simulink model "bldc_cc_2020a"  (R2020a)
settings: Solver=VariableStepAuto  StartTime=0.0  StopTime=10  RelTol=1e-3
undefined symbols (not defined in the file or in its folder): Ion, Lithium
libraries: spsMosfetLib x6, spsSeriesRLCBranchLib x3, simulink x3, spsBatteryLib x1, spsPermanentMagnetSynchronousMachineLib x1, spspowerguiLib x1
settings Model: Creator=Deepak  LastModifiedBy=giulio
settings SFSimCC: CustomCodeUndefinedFunction=UseInterfaceOnly

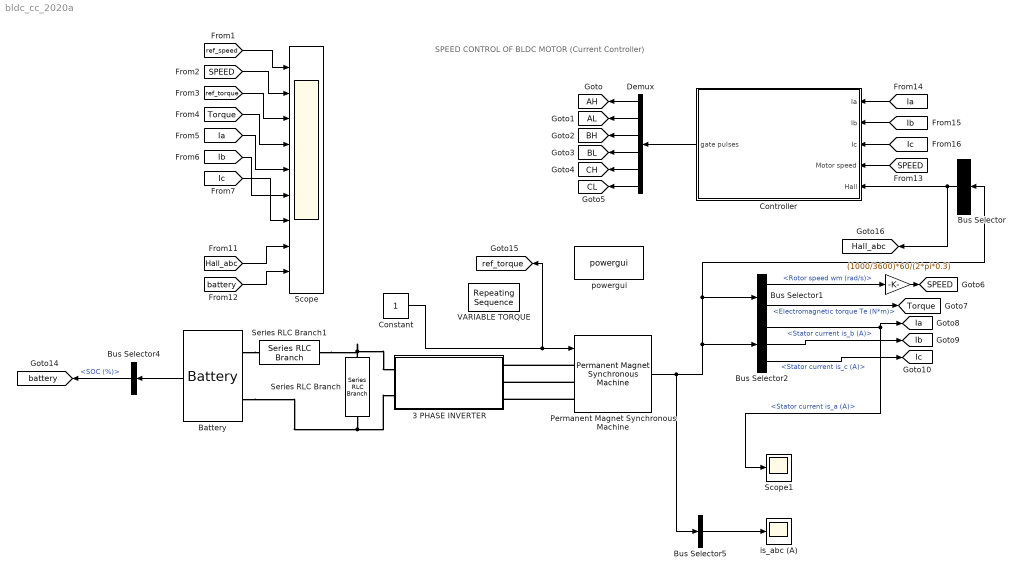
== system bldc_cc_2020a ==
  note: SPEED CONTROL OF BLDC MOTOR (Current Controller)
  " " : Gain  Gain=(1000/3600)*60/(2*pi*0.3)
  3 PHASE INVERTER : Subsystem
  Battery : spsBatteryLib/Battery  BatType=Lithium-Ion  ShowTempParam=off  ThermalPreset=no  ShowAgeParam=off  NomV=12  NomQ=80  SOC=60  Batt_Tr=30  PresetModel=off  MaxQ=84  MinV=36  FullV=56.818272  Dis_rate=27.82608  R=0.006  Normal_OP=57.87524  expZone=[54.89208 3.144344]  current=[1.5 3]  Units=Ampere-hour  Tci=20  NomT=20  T2=-30  MaxQ2=4.8  FullV2=7.1  Normal_OP2=5.655  expZone2="[6.58           1]"  Rca=0.6  ti=2000  Dp=0  Neq0=0  Tsim=1e6  Ta1=25  Qeol=5.4*0.9  Reol=0.013333*1.2  Char_age=[2.3478, 3]  Dis_age=[2.3478, 10]  N1=1500  N2=10500  N3=1000  N4=1400  Ta2=45  N5=950
  Bus Selector : BusSelector  OutputSignals=Hall effect signal h_a,Hall effect signal h_b,Hall effect signal h_c  OutputAsBus=on
  Bus Selector1 : BusSelector  OutputSignals=Rotor speed wm (rad/s),Electromagnetic torque Te (N*m)
  Bus Selector2 : BusSelector  OutputSignals=Stator current is_a (A),Stator current is_b (A),Stator current is_c (A)
  Bus Selector4 : BusSelector  OutputSignals=SOC (%)
  Bus Selector5 : BusSelector  OutputSignals=Stator current is_a (A),Stator current is_b (A),Stator current is_c (A)  OutputAsBus=on
  Constant : Constant
  Controller : Subsystem
  Demux : Demux  Outputs=6
  Permanent Magnet Synchronous Machine : spsPermanentMagnetSynchronousMachineLib/Permanent Magnet Synchronous Machine  NbPhases=3  FluxDistribution=Sinusoidal  RotorType=Round  MechanicalLoad=Torque Tm  PresetModel=No  ShowDetailedParameters=on  MeasurementBus=off  Resistance=2.875  Inductance=8.5e-3  dqInductances=[8.5e-3,8.5e-3]  La=0.00153  MachineConstant=Flux linkage established by magnets (V.s)  Flux=0.175  VoltageCst=126.966  TorqueCst=1.05  Flat=120  Mechanical=[ 0.8e-3, 0 4]  PolePairs=4  InitialConditions=[0,0, 0,0]  InitialConditions5ph=[0 0 0 0 0 0]  RefAngle=90 degrees behind phase A axis (modified Park)  IterativeDiscreteModel=Trapezoidal non iterative  TsBlock=-1  TsPowergui=0
  Scope : Scope  NumInputPorts=9
  Scope1 : Scope
  Series RLC Branch : spsSeriesRLCBranchLib/Series RLC Branch  LConnTagsString=__new0  RConnTagsString=__new0  BranchType=C  Resistance=1  Inductance=1e-3  SetiL0=off  InitialCurrent=0  Capacitance=75e-3  Setx0=off  InitialVoltage=0  Measurements=None
  Series RLC Branch1 : spsSeriesRLCBranchLib/Series RLC Branch  LConnTagsString=__new0  RConnTagsString=__new0  BranchType=RL  Resistance=1  Inductance=1e-3  SetiL0=off  InitialCurrent=0  Capacitance=75e-3  Setx0=off  InitialVoltage=0  Measurements=None
  VARIABLE TORQUE : simulink/Sources/Repeating Sequence  rep_seq_t=[0 1 2 3 4 5 6 7 8 9 10 11 12 13]  rep_seq_y=[3 3 3 3 5 5 5 -2 -2 -2 1 1 1 1 ]
  is_abc (A) : Scope
  powergui : spspowerguiLib/powergui  Priority=1  SimulationMode=Discrete  SampleTime=10e-6  frequency=60  Iterations=50  frequencyindice=0  Pbase=100e6  ErrMax=1e-4  UnitsV=kV  UnitsW=MW  buscounter=0  FunctionMessages=off  echomessages=off  EnableUseOfTLC=off  CurrentSourceSwitches=off  DisableSnubberDevices=off  DisableRonSwitches=off  DisableVfSwitches=off  DisplayEquations=off  AutomaticDiscreteSolvers=off  SolverType=Tustin/Backward Euler (TBE)  Interpol=off  ExternalGateDelay=off  methode=off  Ts=100  x0status=blocks  SPID=on  SwTol=0  HookPort=off  NonlinearTolerance=0  nMaxIteration=15  ContinueOnMaxIteration=off  RestoreLinks=warning  ResistiveCurrentMeasurement=off  Frange=[0:2:500]  Ylog=off  Xlog=on  ShowGrid=off  save=off  variable=ZData  structure=0  ZoomFFT=off  StartTime=0.0  cycles=1  DisplayStyle=1  fundamental=60  FreqAxis=off  MaxFrequency=1000  frequencyindicesteady=1  RmsSteady=1  display=off
  tag scope: AH=global, AL=global, BH=global, BL=global, CH=global, CL=global, Hall_abc=global, Ia=global, Ib=global, Ic=global, SPEED=global, Torque=global, battery=global, ref_torque=global
  wires:
  [SPEED] -> Scope/2
  [ref_torque] -> Scope/3
  [Ic] -> Scope/7
  Bus Selector2/2 -> [Ib]  "<Stator current is_b (A)>"
  [Hall_abc] -> Scope/8
  Demux/4 -> [BL]
  Demux/3 -> [BH]
  " "/1 -> [SPEED]
  [Ib] -> Scope/6
  [Ia] -> Scope/5
  Bus Selector2/3 -> [Ic]  "<Stator current is_c (A)>"
  [Torque] -> Scope/4
  Bus Selector1/1 -> " "/1  "<Rotor speed wm (rad/s)>"
  [battery] -> Scope/9
  Bus Selector1/2 -> [Torque]  "<Electromagnetic torque Te (N*m)>"
  [ref_speed] -> Scope/1
  Demux/5 -> [CH]
  Demux/1 -> [AH]
  Demux/6 -> [CL]
  Demux/2 -> [AL]
  Bus Selector2/1 -> Scope1/1, [Ia]  "<Stator current is_a (A)>"
  Bus Selector/1 -> Controller/5("Hall "), [Hall_abc]
  [SPEED] -> Controller/4(Motor speed)
  [Ia] -> Controller/1(Ia)
  [Ib] -> Controller/2(Ib)
  [Ic] -> Controller/3(Ic)
  Controller/1(gate pulses) -> Demux/1
  Battery/1 -> Bus Selector4/1
  Bus Selector4/1 -> [battery]  "<SOC (%)>"
  Constant/1 -> Permanent Magnet Synchronous Machine/1, [ref_torque]
  Bus Selector5/1 -> is_abc (A)/1
  Permanent Magnet Synchronous Machine/1 -> Bus Selector5/1, Bus Selector/1, Bus Selector1/1, Bus Selector2/1
  connections:
  Permanent Magnet Synchronous Machine/LConn2 -- 3 PHASE INVERTER/RConn2
  Permanent Magnet Synchronous Machine/LConn3 -- 3 PHASE INVERTER/RConn3
  Permanent Magnet Synchronous Machine/LConn1 -- 3 PHASE INVERTER/RConn1
  Battery/LConn2 -- Series RLC Branch/RConn1 -- 3 PHASE INVERTER/LConn2
  Series RLC Branch/LConn1 -- Series RLC Branch1/LConn1 -- 3 PHASE INVERTER/LConn1
  Battery/LConn1 -- Series RLC Branch1/RConn1

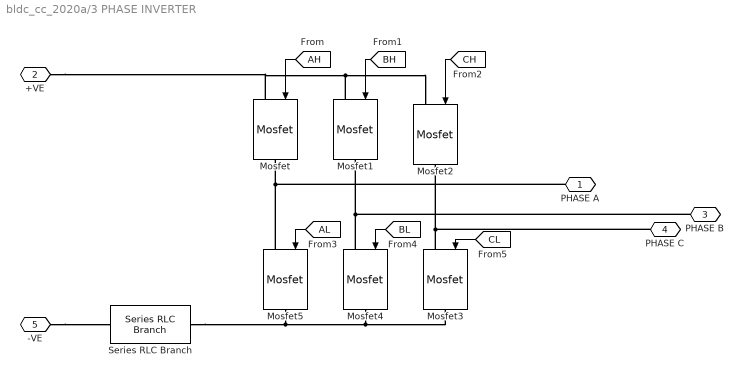
== system bldc_cc_2020a/3 PHASE INVERTER ==
  Mosfet{,1..5} (6 alike) : spsMosfetLib/Mosfet  Ron=0.1  Lon=0  Rd=0.01  Vfd=0  IC=0  Rs=1e5  Cs=inf  Measurements=off
  Series RLC Branch : spsSeriesRLCBranchLib/Series RLC Branch  LConnTagsString=__new0  RConnTagsString=__new0  BranchType=R  Resistance=1  Inductance=1e-3  SetiL0=off  InitialCurrent=0  Capacitance=1e-6  Setx0=off  InitialVoltage=0  Measurements=None
  PHASE A : PMIOPort  Side=Right
  +VE : PMIOPort  Port=2  Side=Left
  PHASE B : PMIOPort  Port=3  Side=Right
  PHASE C : PMIOPort  Port=4  Side=Right
  -VE : PMIOPort  Port=5  Side=Left
  wires:
  [AH] -> Mosfet/1
  [BH] -> Mosfet1/1
  [CH] -> Mosfet2/1
  [AL] -> Mosfet5/1
  [BL] -> Mosfet4/1
  [CL] -> Mosfet3/1
  connections:
  Mosfet5/LConn1 -- PHASE A/RConn1 -- Mosfet/RConn1
  PHASE B/RConn1 -- Mosfet4/LConn1 -- Mosfet1/RConn1
  Mosfet3/LConn1 -- Mosfet2/RConn1 -- PHASE C/RConn1
  Mosfet1/LConn1 -- Mosfet2/LConn1 -- Mosfet/LConn1 -- +VE/RConn1
  Mosfet5/RConn1 -- Series RLC Branch/RConn1 -- Mosfet4/RConn1 -- Mosfet3/RConn1
  -VE/RConn1 -- Series RLC Branch/LConn1

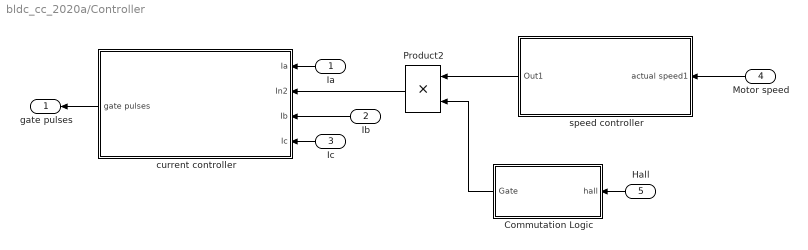
== system bldc_cc_2020a/Controller ==
  Ia : Inport
  Ib : Inport  Port=2
  Ic : Inport  Port=3
  Motor speed : Inport  Port=4
  "Hall " : Inport  Port=5
  Commutation Logic : Subsystem
  Product2 : Product  SaturateOnIntegerOverflow=on  OutDataTypeStr=Inherit: Same as first input
  current controller : Subsystem
  speed controller : Subsystem
  gate pulses : Outport  VectorParamsAs1DForOutWhenUnconnected=off
  wires:
  "Hall "/1 -> Commutation Logic/1("hall ")
  Commutation Logic/1(Gate) -> Product2/2
  current controller/1(gate pulses) -> gate pulses/1
  Ic/1 -> current controller/4(Ic)
  Ib/1 -> current controller/3(Ib)
  Ia/1 -> current controller/1(Ia)
  Product2/1 -> current controller/2(In2)
  Motor speed/1 -> speed controller/1(actual speed1)
  speed controller/1(Out1) -> Product2/1

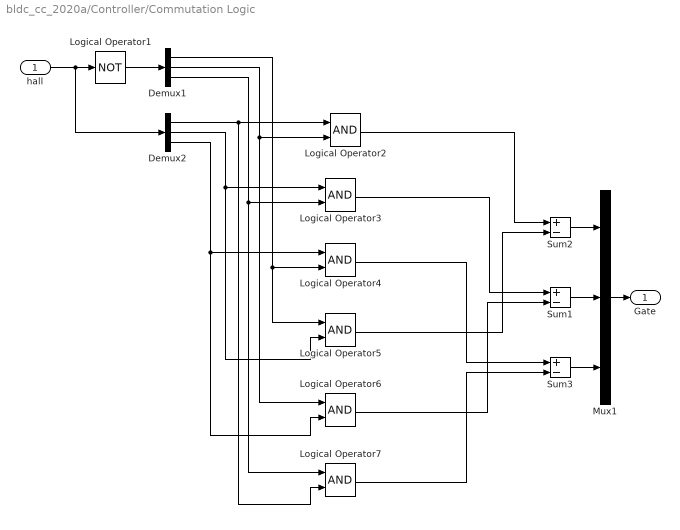
== system bldc_cc_2020a/Controller/Commutation Logic ==
  "hall " : Inport
  Demux1 : Demux  Outputs=3
  Demux2 : Demux  Outputs=3
  Logical Operator1 : Logic  Operator=NOT  AllPortsSameDT=off  OutDataTypeStr=boolean
  Logical Operator{2..7} (6 alike) : Logic  AllPortsSameDT=off  OutDataTypeStr=boolean
  Mux1 : Mux  Inputs=3
  Sum1 : Sum  Inputs=+-  OutDataTypeStr=double
  Sum2 : Sum  Inputs=+-  OutDataTypeStr=double
  Sum3 : Sum  Inputs=+-  OutDataTypeStr=double
  Gate : Outport  VectorParamsAs1DForOutWhenUnconnected=off
  wires:
  Demux2/1 -> Logical Operator7/2, Logical Operator2/1
  Demux1/3 -> Logical Operator7/1, Logical Operator3/2
  Demux2/2 -> Logical Operator3/1, Logical Operator5/2
  Sum1/1 -> Mux1/2
  Logical Operator3/1 -> Sum1/1
  "hall "/1 -> Logical Operator1/1, Demux2/1
  Demux1/2 -> Logical Operator6/1, Logical Operator2/2
  Logical Operator2/1 -> Sum2/1
  Logical Operator7/1 -> Sum3/2
  Logical Operator4/1 -> Sum3/1
  Demux1/1 -> Logical Operator4/2, Logical Operator5/1
  Logical Operator6/1 -> Sum1/2
  Logical Operator5/1 -> Sum2/2
  Sum3/1 -> Mux1/3
  Logical Operator1/1 -> Demux1/1
  Mux1/1 -> Gate/1
  Sum2/1 -> Mux1/1
  Demux2/3 -> Logical Operator4/1, Logical Operator6/2

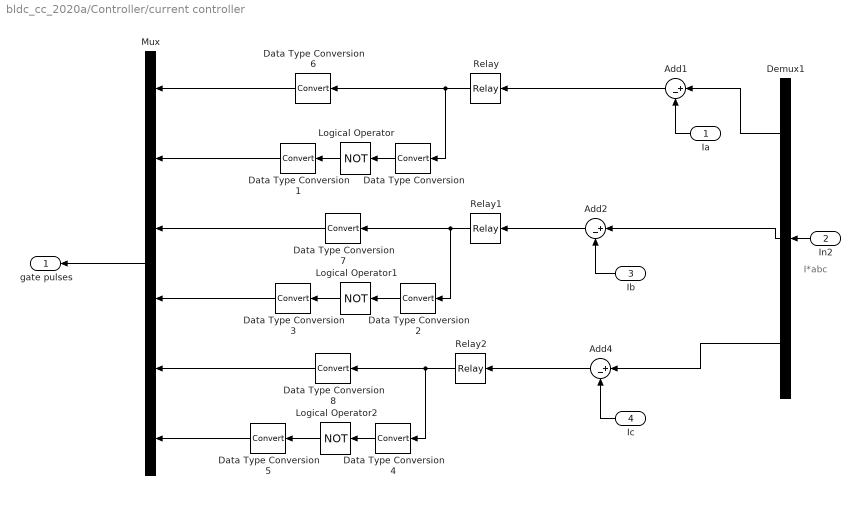
== system bldc_cc_2020a/Controller/current controller ==
  note: I*abc
  Ia : Inport
  In2 : Inport  Port=2
  Ib : Inport  Port=3
  Ic : Inport  Port=4
  Add1 : Sum  Inputs=|+-
  Add2 : Sum  Inputs=|+-
  Add4 : Sum  Inputs=|+-
  Data Type Conversion{,1..8} (9 alike) : DataTypeConversion  SaturateOnIntegerOverflow=on  RndMeth=Zero
  Demux1 : Demux  Outputs=3
      settings: DisplayOption=none
  Logical Operator : Logic  Operator=NOT  AllPortsSameDT=off  OutDataTypeStr=boolean
  Logical Operator1 : Logic  Operator=NOT  AllPortsSameDT=off  OutDataTypeStr=boolean
  Logical Operator2 : Logic  Operator=NOT  AllPortsSameDT=off  OutDataTypeStr=boolean
  Mux : Mux  Inputs=6
  Relay : Relay  OnSwitchValue=0.1  OffSwitchValue=-0.1
  Relay1 : Relay  OnSwitchValue=0.1  OffSwitchValue=-0.1
  Relay2 : Relay  OnSwitchValue=0.1  OffSwitchValue=-0.1
  gate pulses : Outport  VectorParamsAs1DForOutWhenUnconnected=off
  wires:
  Relay/1 -> Data Type Conversion6/1, Data Type Conversion/1
  Relay1/1 -> Data Type Conversion7/1, Data Type Conversion2/1
  Relay2/1 -> Data Type Conversion8/1, Data Type Conversion4/1
  Ib/1 -> Add2/2
  Mux/1 -> gate pulses/1
  Ic/1 -> Add4/2
  Data Type Conversion/1 -> Logical Operator/1
  Logical Operator/1 -> Data Type Conversion1/1
  Data Type Conversion1/1 -> Mux/2
  Logical Operator1/1 -> Data Type Conversion3/1
  Data Type Conversion3/1 -> Mux/4
  Data Type Conversion2/1 -> Logical Operator1/1
  Data Type Conversion5/1 -> Mux/6
  Logical Operator2/1 -> Data Type Conversion5/1
  Data Type Conversion4/1 -> Logical Operator2/1
  Demux1/2 -> Add2/1
  Demux1/3 -> Add4/1
  In2/1 -> Demux1/1
  Ia/1 -> Add1/2
  Demux1/1 -> Add1/1
  Add1/1 -> Relay/1
  Add2/1 -> Relay1/1
  Data Type Conversion6/1 -> Mux/1
  Data Type Conversion7/1 -> Mux/3
  Data Type Conversion8/1 -> Mux/5
  Add4/1 -> Relay2/1

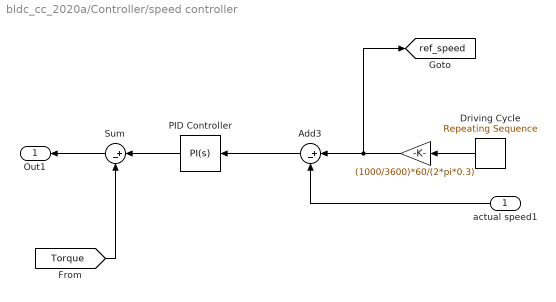
== system bldc_cc_2020a/Controller/speed controller ==
  actual speed1 : Inport
  " " : Gain  Gain=(1000/3600)*60/(2*pi*0.3)
  Add3 : Sum  Inputs=|+-
  Driving Cycle : simulink/Sources/Repeating Sequence  rep_seq_t=[0 1 2 3 4 5 6 7 8 9 10 11 11.0001 12 13]  rep_seq_y=[0 0 20 20 20 20 20 20 20 20 20 20 20 20 20]
  PID Controller : simulink/Continuous/PID Controller  Controller=PI  Form=Parallel  TimeDomain=Continuous-time  UseExternalTs=off  SampleTime=-1  IntegratorMethod=Forward Euler  FilterMethod=Forward Euler  ControllerParametersSource=internal  P=5  I=4.9  D=0  UseFilter=on  N=100  TunerSelectOption=Transfer Function Based (PID Tuner App)  InitialConditionSource=internal  InitialConditionForIntegrator=0  InitialConditionForFilter=0  DifferentiatorICPrevScaledInput=0  ExternalReset=none  TrackingMode=off  Kt=1  LimitOutput=off  UpperSaturationLimit=10  LowerSaturationLimit=0  LinearizeAsGain=on  AntiWindupMode=none  Kb=1  POutMin=[]  POutMax=[]  IOutMin=[]  IOutMax=[]  DOutMin=[]  DOutMax=[]  NOutMin=[]  NOutMax=[]  SumOutMin=[]  SumOutMax=[]  SaturationOutMin=[]  SaturationOutMax=[]  PParamMin=[]  PParamMax=[]  IParamMin=[]  IParamMax=[]  DParamMin=[]  DParamMax=[]  NParamMin=[]  NParamMax=[]  KbParamMin=[]  KbParamMax=[]  KtParamMin=[]  KtParamMax=[]  KbOutMin=[]  KbOutMax=[]  KtOutMin=[]  KtOutMax=[]  IntegratorOutMin=[]  IntegratorOutMax=[]  FilterOutMin=[]  FilterOutMax=[]  SumI1OutMin=[]  SumI1OutMax=[]  SumI2OutMin=[]  SumI2OutMax=[]  SumI3OutMin=[]  SumI3OutMax=[]  SumI4OutMin=[]  SumI4OutMax=[]  SumDOutMin=[]  SumDOutMax=[]  DifferentiatorOutMin=[]  DifferentiatorOutMax=[]  FilterDiffOutCoefMin=[]  FilterDiffOutCoefMax=[]  ReciprocalOutMin=[]  ReciprocalOutMax=[]  SumDenOutMin=[]  SumDenOutMax=[]  SumNumOutMin=[]  SumNumOutMax=[]  DivideOutMin=[]  DivideOutMax=[]  UdiffTsProdOutMin=[]  UdiffTsProdOutMax=[]  NTsProdOutMin=[]  NTsProdOutMax=[]  UintegralTsProdOutMin=[]  UintegralTsProdOutMax=[]  UngainTsProdOutMin=[]  UngainTsProdOutMax=[]  IntegratorContinuousStateAttributes=''  IntegratorStateMustResolveToSignalObject=off  IntegratorRTWStateStorageClass=Auto  FilterContinuousStateAttributes=''  FilterStateMustResolveToSignalObject=off  FilterRTWStateStorageClass=Auto  ParallelPVariant=InternalParameters  IdealPVariant=Disabled  IVariant=InternalParameters  DVariant=Disabled  IntegratorVariant=Continuous  SatVariant=Disabled  AWVariant=Passthrough  PCopyVariant=Disabled  TRVariant=Disabled  FdbkBlocksVariant=Forward  IdealPFdbkVariant=Disabled  SatFdbkVariant=Disabled  DerivativeFilterVariant=Disabled  NVariant=Disabled  NCopyVariant=Disabled_SignalSpec  FilterICVariant=Disabled  IntegratorICVariant=InternalICs  ExternalResetVariant=Disabled  TRSumVariant=Passthrough  SumFdbkVariant=Disabled  SumVariant=Sum_PI  TsampFilterVariant=InternalTs  TsampNgainVariant=Passthrough  TsampIntegralVariant=Passthrough
  Sum : Sum  Inputs=|+-
  Out1 : Outport  VectorParamsAs1DForOutWhenUnconnected=off
  tag scope: ref_speed=global
  wires:
  Add3/1 -> PID Controller/1
  actual speed1/1 -> Add3/2
  PID Controller/1 -> Sum/1
  [Torque] -> Sum/2
  Sum/1 -> Out1/1
  " "/1 -> [ref_speed], Add3/1
  Driving Cycle/1 -> " "/1
